simulink model "Controllo_Ottimo_LQ"  (R2023b)
settings: Solver=VariableStepAuto  StartTime=0.0  StopTime=50  RelTol=1e-3
undefined symbols (not defined in the file): A, A_obs, B, B_obs, C, C_obs, D, D_obs, Fi, Fr
settings Model: Creator=emman  LastModifiedBy=emman

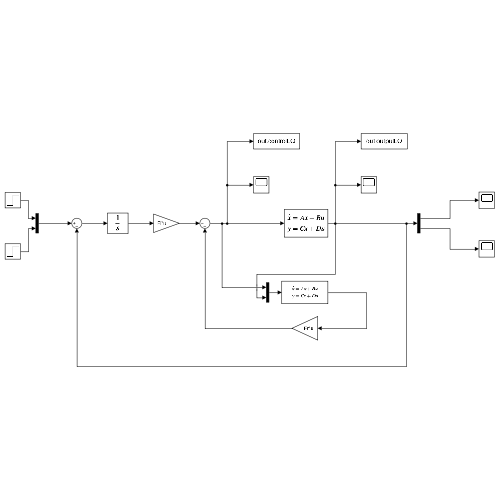
[thumbnail: Simulink's stored preview of the top-level diagram]
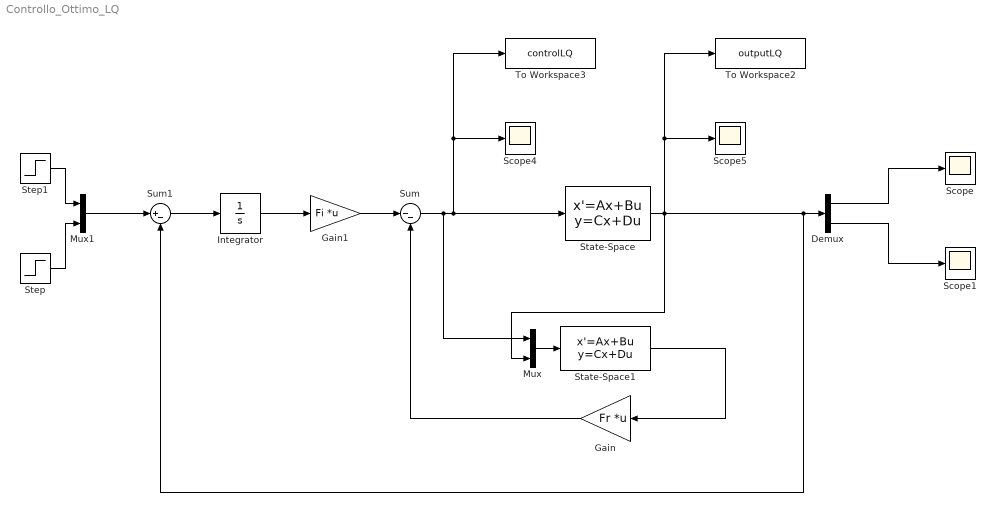
== system Controllo_Ottimo_LQ ==
  Demux : Demux  Outputs=2
  Gain : Gain  Gain=Fr  Multiplication=Matrix(K*u)
  Gain1 : Gain  Gain=Fi  Multiplication=Matrix(K*u)
  Integrator : Integrator
  Mux : Mux  Inputs=2
  Mux1 : Mux  Inputs=2
  Scope{,1,4..5} (4 alike) : Scope
  State-Space : StateSpace  A=A  B=B  C=C  D=D  InitialCondition=0  ParameterTunability=Unconstrained
  State-Space1 : StateSpace  A=A_obs  B=B_obs  C=C_obs  D=D_obs  InitialCondition=0
  Step : Step  Time=0  After=2.5  SampleTime=0
  Step1 : Step  Time=0  After=2  SampleTime=0
  Sum : Sum  Inputs=|--
  Sum1 : Sum  Inputs=|+-
  To Workspace2 : ToWorkspace  VariableName=outputLQ  SaveFormat=Structure With Time  SampleTime=-1
  To Workspace3 : ToWorkspace  VariableName=controlLQ  SaveFormat=Structure With Time  SampleTime=-1
  wires:
  Gain/1 -> Sum/2
  State-Space1/1 -> Gain/1
  Step1/1 -> Mux1/1
  Demux/1 -> Scope/1
  Mux/1 -> State-Space1/1
  Integrator/1 -> Gain1/1
  State-Space/1 -> To Workspace2/1, Scope5/1, Sum1/2, Demux/1, Mux/2
  Sum1/1 -> Integrator/1
  Mux1/1 -> Sum1/1
  Step/1 -> Mux1/2
  Demux/2 -> Scope1/1
  Sum/1 -> Scope4/1, To Workspace3/1, State-Space/1, Mux/1
  Gain1/1 -> Sum/1
